simulink model "SpringMassSystem"  (R2024a)
settings: Solver=ode45  StartTime=0.0  StopTime=10.0  RelTol=1e-10
settings Model: Creator=tristan  LastModifiedBy=tristan

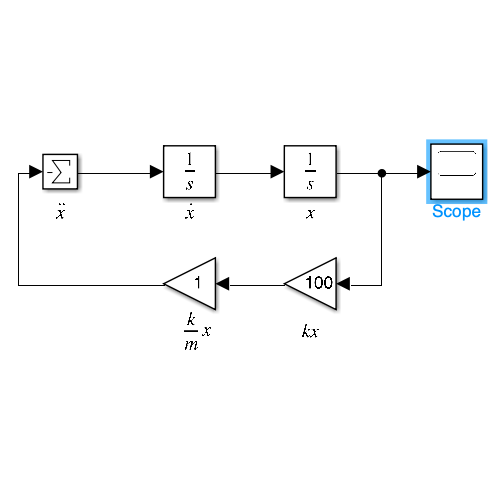
[thumbnail: Simulink's stored preview of the top-level diagram]
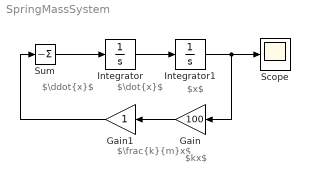
== system SpringMassSystem ==
  note: $\frac{k}{m}x$
  note: $kx$
  note: $x$
  note: $\ddot{x}$
  note: $\dot{x}$
  Gain : Gain  Gain=100
  Gain1 : Gain
  Integrator : Integrator
  Integrator1 : Integrator  InitialCondition=1
  Scope : Scope
  Sum : Sum  Inputs=-
  wires:
  Sum/1 -> Integrator/1
  Integrator/1 -> Integrator1/1
  Integrator1/1 -> Scope/1, Gain/1
  Gain/1 -> Gain1/1
  Gain1/1 -> Sum/1
